simulink model "FRUCDVehicleModel"  (R2020b)
settings: Solver=VariableStepAuto  StartTime=0.0  StopTime=10.0  RelTol=1e-3
undefined symbols (not defined in the file): Vehicle, zero
settings Model: Creator=Authorized User  LastModifiedBy=Authorized User

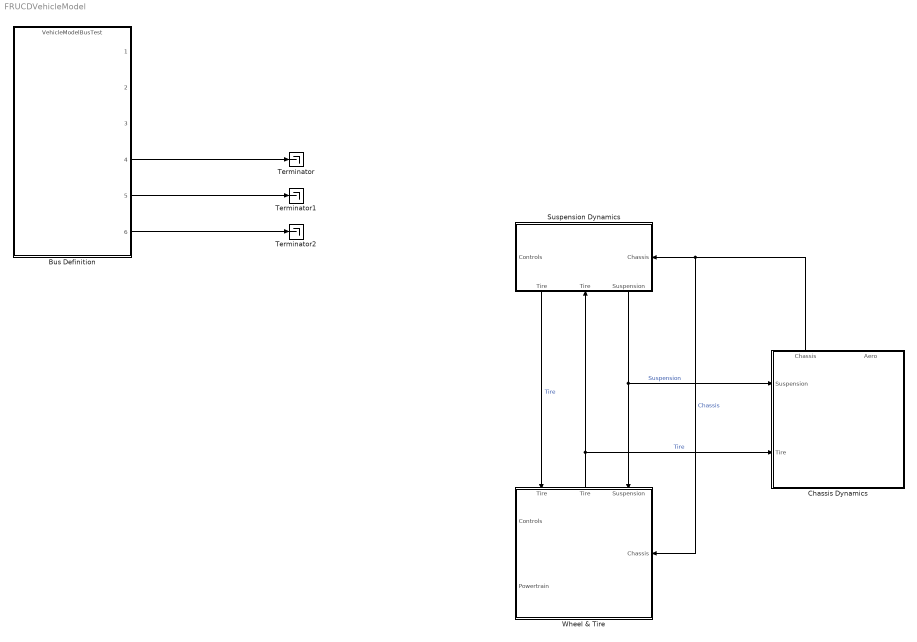
== system FRUCDVehicleModel ==
  Bus Definition : ModelReference  ModelNameDialog=VehicleModelBusTest.slx  SimulationMode=Normal  ModelReferenceVersion=1.33
  Chassis Dynamics : Subsystem  Variant=on
      settings: PortSchema="{\"entries\":[{\"content\":{\"sides\":[{\"content\":{\"connectorIds\":[\"In1\",\"In2\"]},\"type\":\"ConnectorPlacement.EquallySpacedRectSide\",\"uuid\":\"401103c9-df33-4d23-92c4-dccc68bb9aee\"},{\"content\":{\"connectorIds\":[],\"side\":\"RIGHT\"},\"type\":\"ConnectorPlacement.EquallySpacedRectSide\",\"uuid\":\"29401883-02eb-405e-b55e-d775bdf22a7d\"},{\"content\":{\"connectorIds\":[\"Out1\",\"In3\"],\"side\":\"TOP\"},\"type\":\"ConnectorPlacement.EquallySpacedRectSide\",\"uuid\":\"28f0344c-81b9-4726-876b-7ae633e27a22\"},{\"content\":{\"connectorIds\":[],\"side\":\"HIDDEN\"},\"type\":\"ConnectorPlacement.EquallySpacedRectSide\",\"uuid\":\"b9c547a4-039e-4e66-a34f-1f08b2b53ac3\"}]},\"type\":\"ConnectorPlacement.EquallySpacedConnector\",\"uuid\":\"813f49e5-5549-40bc-88e7-d74b73b169a6\"}],\"packageUris\":[\"http://schema.mathworks.com/mf0/Connector/R2020b\"],\"version\":\"1.0\"}"
  Suspension Dynamics : Subsystem  Variant=on
      settings: PortSchema="{\"entries\":[{\"content\":{\"sides\":[{\"content\":{\"connectorIds\":[\"In1\"]},\"type\":\"ConnectorPlacement.EquallySpacedRectSide\",\"uuid\":\"ac39668b-b0ed-403b-8381-303be083bc77\"},{\"content\":{\"connectorIds\":[\"In3\"],\"side\":\"RIGHT\"},\"type\":\"ConnectorPlacement.EquallySpacedRectSide\",\"uuid\":\"f6b1d0bd-c35b-44a1-b6f6-628e84c5d84e\"},{\"content\":{\"connectorIds\":[],\"side\":\"TOP\"},\"type\":\"ConnectorPlacement.EquallySpacedRectSide\",\"uuid\":\"82d42e0f-c7c6-4998-bfd6-14096c24fb9e\"},{\"content\":{\"connectorIds\":[\"Out1\",\"In2\",\"Out2\"],\"side\":\"BOTTOM\"},\"type\":\"ConnectorPlacement.EquallySpacedRectSide\",\"uuid\":\"c47917f9-6923-47fe-90c8-09706c27f893\"},{\"content\":{\"connectorIds\":[],\"side\":\"HIDDEN\"},\"type\":\"ConnectorPlacement.EquallySpacedRectSide\",\"uuid\":\"da3a1ff4-a909-4137-bdfb-403e7529f4b5\"}]},\"type\":\"ConnectorPlacement.EquallySpacedConnector\",\"uuid\":\"02c616f2-d1b9-4bce-afea-494318e317d7\"}],\"packageUris\":[\"http://schema.mathworks.com/mf0/Connector/R2020b\"],\"version\":\"1.0\"}"
      mask Display: image('C:\Users\Authorized User\Downloads\FSAE Suspension.jpg'); % Use "Edit Image" on toolstrip to change.
  Terminator : Terminator
  Terminator1 : Terminator
  Terminator2 : Terminator
  Wheel & Tire : Subsystem
      settings: PortSchema="{\"entries\":[{\"content\":{\"sides\":[{\"content\":{\"connectorIds\":[\"In1\",\"In2\"]},\"type\":\"ConnectorPlacement.EquallySpacedRectSide\",\"uuid\":\"ac39668b-b0ed-403b-8381-303be083bc77\"},{\"content\":{\"connectorIds\":[\"In5\"],\"side\":\"RIGHT\"},\"type\":\"ConnectorPlacement.EquallySpacedRectSide\",\"uuid\":\"f6b1d0bd-c35b-44a1-b6f6-628e84c5d84e\"},{\"content\":{\"connectorIds\":[\"In3\",\"Out1\",\"In4\"],\"side\":\"TOP\"},\"type\":\"ConnectorPlacement.EquallySpacedRectSide\",\"uuid\":\"82d42e0f-c7c6-4998-bfd6-14096c24fb9e\"},{\"content\":{\"connectorIds\":[],\"side\":\"HIDDEN\"},\"type\":\"ConnectorPlacement.EquallySpacedRectSide\",\"uuid\":\"da3a1ff4-a909-4137-bdfb-403e7529f4b5\"}]},\"type\":\"ConnectorPlacement.EquallySpacedConnector\",\"uuid\":\"02c616f2-d1b9-4bce-afea-494318e317d7\"}],\"packageUris\":[\"http://schema.mathworks.com/mf0/Connector/R2020b\"],\"version\":\"1.0\"}"
  wires:
  Bus Definition/5 -> Terminator1/1
  Bus Definition/4 -> Terminator/1
  Bus Definition/6 -> Terminator2/1
  Suspension Dynamics/2("Suspension ") -> Chassis Dynamics/1(Suspension), Wheel & Tire/4(Suspension)  "Suspension"
  Suspension Dynamics/1("Tire ") -> Wheel & Tire/3(Tire)  "Tire"
  Wheel & Tire/1("Tire ") -> Chassis Dynamics/2(Tire), Suspension Dynamics/2(Tire)  "Tire"
  Chassis Dynamics/1(Chassis) -> Suspension Dynamics/3(Chassis), Wheel & Tire/5(Chassis)  "Chassis"

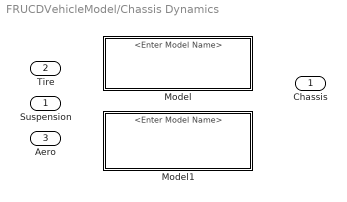
== system FRUCDVehicleModel/Chassis Dynamics ==
  Suspension : Inport
  Tire : Inport  Port=2
  Aero : Inport  Port=3
  Model : ModelReference  DisableCoverage=on  VariantControl=Variant
  Model1 : ModelReference  VariantControl=Variant1
  Chassis : Outport

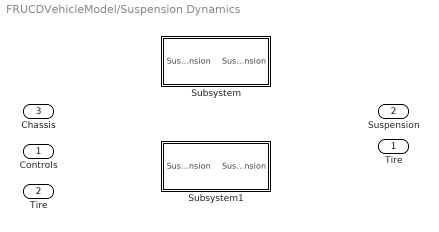
== system FRUCDVehicleModel/Suspension Dynamics ==
  Controls : Inport
  Tire : Inport  Port=2
  Chassis : Inport  Port=3
  Subsystem : Subsystem  VariantControl=Choice_1
  Subsystem1 : Subsystem  VariantControl=Choice_2
  "Tire " : Outport
  "Suspension " : Outport  Port=2

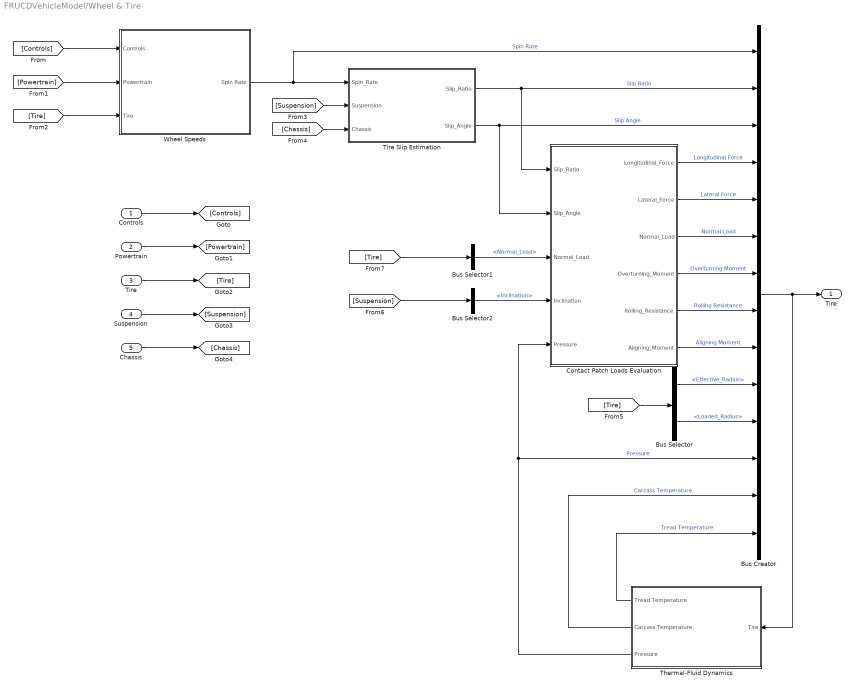
== system FRUCDVehicleModel/Wheel & Tire ==
  Controls : Inport  OutDataTypeStr=Bus: Controls
  Powertrain : Inport  Port=2  OutDataTypeStr=Bus: Powertrain
  Tire : Inport  Port=3  OutDataTypeStr=Bus: Tire
  Suspension : Inport  Port=4  OutDataTypeStr=Bus: Suspension
  Chassis : Inport  Port=5  OutDataTypeStr=Bus: Chassis
  Bus Creator : BusCreator  Inputs=14
  Bus Selector : BusSelector  OutputSignals=Effective_Radius,Loaded_Radius
  Bus Selector1 : BusSelector  OutputSignals=Normal_Load
  Bus Selector2 : BusSelector  OutputSignals=Inclination
  Contact Patch Loads Evaluation : MATLAB Function  TreatAsAtomicUnit=on
  Thermal-Fluid Dynamics : Subsystem  Variant=on
  Tire Slip Estimation : MATLAB Function  TreatAsAtomicUnit=on
  Wheel Speeds : Subsystem
  "Tire " : Outport  OutDataTypeStr=Bus: Tire
  wires:
  Tire Slip Estimation/2(Slip_Angle) -> Contact Patch Loads Evaluation/2(Slip_Angle), Bus Creator/3  "Slip Angle"
  Tire Slip Estimation/1(Slip_Ratio) -> Contact Patch Loads Evaluation/1(Slip_Ratio), Bus Creator/2  "Slip Ratio"
  Bus Creator/1 -> "Tire "/1, Thermal-Fluid Dynamics/1(Tire)
  Wheel Speeds/1(Spin Rate) -> Tire Slip Estimation/1(Spin_Rate), Bus Creator/1  "Spin Rate"
  Contact Patch Loads Evaluation/3(Normal_Load) -> Bus Creator/6  "Normal Load"
  Contact Patch Loads Evaluation/4(Overturning_Moment) -> Bus Creator/7  "Overturning Moment"
  Contact Patch Loads Evaluation/1(Longitudinal_Force) -> Bus Creator/4  "Longitudinal Force"
  Contact Patch Loads Evaluation/5(Rolling_Resistance) -> Bus Creator/8  "Rolling Resistance"
  Contact Patch Loads Evaluation/2(Lateral_Force) -> Bus Creator/5  "Lateral Force"
  Contact Patch Loads Evaluation/6(Aligning_Moment) -> Bus Creator/9  "Aligning Moment"
  Suspension/1 -> [Suspension]
  Tire/1 -> [Tire]
  Powertrain/1 -> [Powertrain]
  Controls/1 -> [Controls]
  Chassis/1 -> [Chassis]
  [Controls] -> Wheel Speeds/1(Controls)
  [Powertrain] -> Wheel Speeds/2(Powertrain)
  [Tire] -> Wheel Speeds/3(Tire)
  [Suspension] -> Tire Slip Estimation/2(Suspension)
  [Chassis] -> Tire Slip Estimation/3(Chassis)
  Bus Selector/1 -> Bus Creator/10  "<Effective_Radius>"
  Bus Selector/2 -> Bus Creator/11  "<Loaded_Radius>"
  Thermal-Fluid Dynamics/3(Pressure) -> Bus Creator/12, Contact Patch Loads Evaluation/5(Pressure)  "Pressure"
  Thermal-Fluid Dynamics/2(Carcass Temperature) -> Bus Creator/13  "Carcass Temperature"
  Thermal-Fluid Dynamics/1(Tread Temperature) -> Bus Creator/14  "Tread Temperature"
  [Tire] -> Bus Selector/1
  [Suspension] -> Bus Selector2/1
  Bus Selector2/1 -> Contact Patch Loads Evaluation/4(Inclination)  "<Inclination>"
  Bus Selector1/1 -> Contact Patch Loads Evaluation/3("Normal_Load ")  "<Normal_Load>"
  [Tire] -> Bus Selector1/1

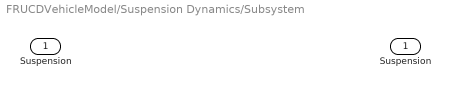
== system FRUCDVehicleModel/Suspension Dynamics/Subsystem ==
  Suspension : Inport
  "Suspension " : Outport

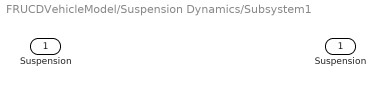
== system FRUCDVehicleModel/Suspension Dynamics/Subsystem1 ==
  Suspension : Inport
  "Suspension " : Outport

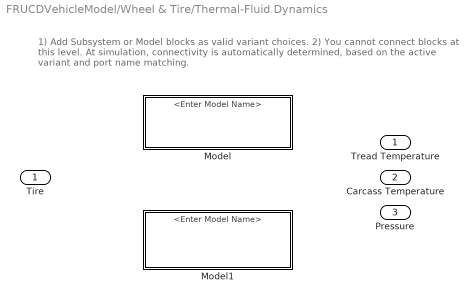
== system FRUCDVehicleModel/Wheel & Tire/Thermal-Fluid Dynamics ==
  note: 1) Add Subsystem or Model blocks as valid variant choices.
      | 2) You cannot connect blocks at this level. At simulation, connectivity is automatically
      | determined, based on the active variant and port name matching.
  Tire : Inport
  Model : ModelReference  DisableCoverage=on  VariantControl=Variant
  Model1 : ModelReference  VariantControl=Variant1
  Tread Temperature : Outport
  Carcass Temperature : Outport  Port=2
  Pressure : Outport  Port=3

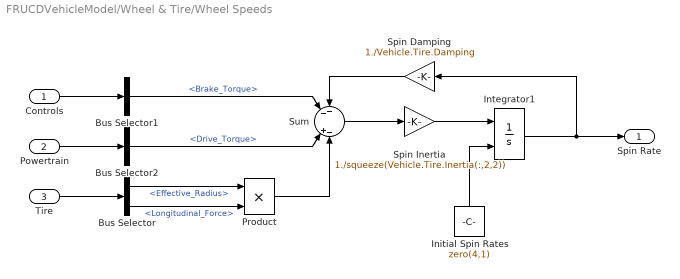
== system FRUCDVehicleModel/Wheel & Tire/Wheel Speeds ==
  Controls : Inport
  Powertrain : Inport  Port=2
  Tire : Inport  Port=3
  Bus Selector : BusSelector  OutputSignals=Effective_Radius,Longitudinal_Force
  Bus Selector1 : BusSelector  OutputSignals=Brake_Torque
  Bus Selector2 : BusSelector  OutputSignals=Drive_Torque
  Initial Spin Rates : Constant  Value=zero(4,1)
  Integrator1 : Integrator  InitialConditionSource=external
  Product : Product
  Spin Damping : Gain  Gain=1./Vehicle.Tire.Damping
  Spin Inertia : Gain  Gain=1./squeeze(Vehicle.Tire.Inertia(:,2,2))
  Sum : Sum  Inputs=--||+-
  Spin Rate : Outport
  wires:
  Spin Damping/1 -> Sum/1
  Sum/1 -> Spin Inertia/1
  Bus Selector2/1 -> Sum/3  "<Drive_Torque>"
  Spin Inertia/1 -> Integrator1/1
  Product/1 -> Sum/4
  Controls/1 -> Bus Selector1/1
  Bus Selector1/1 -> Sum/2  "<Brake_Torque>"
  Bus Selector/1 -> Product/1  "<Effective_Radius>"
  Bus Selector/2 -> Product/2  "<Longitudinal_Force>"
  Integrator1/1 -> Spin Damping/1, Spin Rate/1
  Powertrain/1 -> Bus Selector2/1
  Tire/1 -> Bus Selector/1
  Initial Spin Rates/1 -> Integrator1/2

== matlab function FRUCDVehicleModel/Wheel & Tire/Contact Patch Loads Evaluation ==
  data: Longitudinal_Force output; Slip_Ratio input; Lateral_Force output; Slip_Angle input; Normal_Load input; Inclination input; Pressure input; Vehicle parameter; Normal_Load output; Overturning_Moment output; Rolling_Resistance output; Aligning_Moment output
function [Longitudinal_Force, Lateral_Force, Normal_Load, ...
    Overturning_Moment, Rolling_Resistance, Aligning_Moment] = ...
    ContactPatchLoads(Slip_Ratio, Slip_Angle, Normal_Load, Inclination, Pressure, Vehicle)

for i = 1:4
   
end

== matlab function FRUCDVehicleModel/Wheel & Tire/Tire Slip Estimation ==
  data: Slip_Ratio output; Spin_Rate input; Slip_Angle output; Suspension input; Chassis input; Vehicle parameter
function [Slip_Ratio, Slip_Angle] = TireSlipEstimation(Spin_Rate, Suspension, Chassis, Vehicle)

Slip_Angle = zeros(4,1);
Slip_Angle(1) = Suspension.Steer(1) - atan2d( (Chassis.Lateral(2) + Vehicle.Chassis.a*Chassis.Yaw(2) ), ...
    ( Chassis.Longitudinal(2) - (Suspension.Track(1)/2)*Chassis.Yaw(2) ) );
Slip_Angle(2) = Suspension.Steer(2) - atan2d( (Chassis.Lateral(2) + Vehicle.Chassis.a*Chassis.Yaw(2) ), ...
    ( Chassis.Longitudinal(2) + (Suspension.Track(2)/2)*Chassis.Yaw(2) ) );
Slip_Angle(3) = Suspension.Steer(3) - atan2d( (Chassis.Lateral(2) - Vehicle.Chassis.b*Chassis.Yaw(2) ), ...
    ( Chassis.Longitudinal(2) - (Suspension.Track(3)/2)*Chassis.Yaw(2) ) );
Slip_Angle(4) = Suspension.Steer(4) - atan2d( (Chassis.Lateral(2) - Vehicle.Chassis.b*Chassis.Yaw(2) ), ...
    ( Chassis.Longitudinal(2) + (Suspension.Track(4)/2)*Chassis.Yaw(2) ) );

v = zeros(4,1);
v(1) = sqrt( ( Chassis.Longitudinal(2) - (Suspension.Track(1)/2)*Chassis.Yaw(2) )^2 + ...
    (Chassis.Lateral(2) + Vehicle.Chassis.a*Chassis.Yaw(2) )^2 );
v(2) = sqrt( ( Chassis.Longitudinal(2) + (Suspension.Track(2)/2)*Chassis.Yaw(2) )^2 + ...
    (Chassis.Lateral(2) + Vehicle.Chassis.a*Chassis.Yaw(2) )^2 );
v(3) = sqrt( ( Chassis.Longitudinal(2) - (Suspension.Track(3)/2)*Chassis.Yaw(2) )^2 + ...
    (Chassis.Lateral(2) - Vehicle.Chassis.b*Chassis.Yaw(2) )^2 );
v(4) = sqrt( ( Chassis.Longitudinal(2) + (Suspension.Track(4)/2)*Chassis.Yaw(2) )^2 + ...
    (Chassis.Lateral(2) - Vehicle.Chassis.b*Chassis.Yaw(2) )^2 );

Slip_Ratio = zeros(4,1);
Slip_Ratio(1) = ( Spin_Rate(1) .* Tire.Effective_Radius ) / ( v(1) .* cosd(Slip_Angle(1)) ) - 1;  
Slip_Ratio(2) = ( Spin_Rate(2) .* Tire.Effective_Radius ) / ( v(2) .* cosd(Slip_Angle(2)) ) - 1;  
Slip_Ratio(3) = ( Spin_Rate(3) .* Tire.Effective_Radius ) / ( v(3) .* cosd(Slip_Angle(3)) ) - 1;  
Slip_Ratio(4) = ( Spin_Rate(4) .* Tire.Effective_Radius ) / ( v(4) .* cosd(Slip_Angle(4)) ) - 1;
